simulink model "switchmodel"  (R2019a)
settings: Solver=FixedStepAuto  StartTime=0.0  StopTime=50  FixedStep=1  RelTol=1e-3
settings Model: Creator=anton  LastModifiedBy=anton

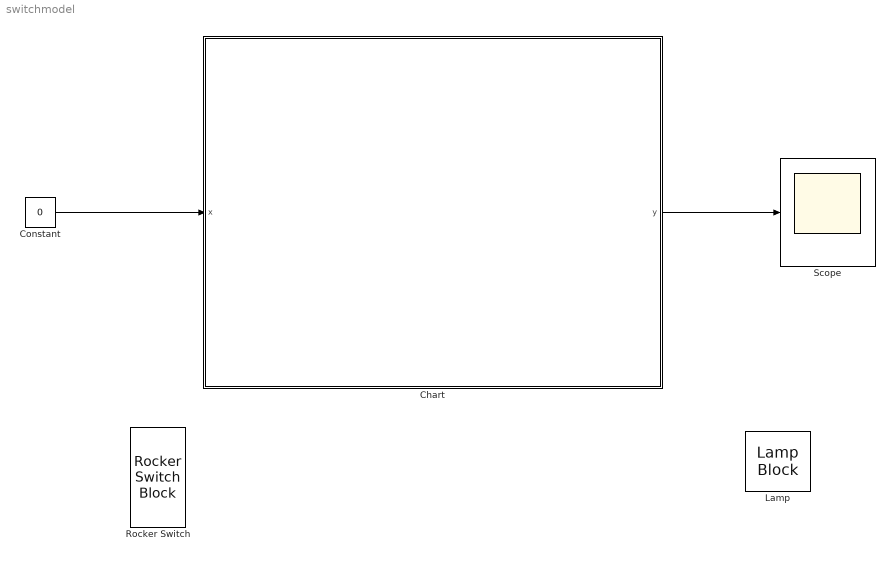
== system switchmodel ==
  Chart : Stateflow chart  BlockKeywords=__PRM__SERIALIZED__DATA__:Stateflow Chart,Stateflow Diagram  TreatAsAtomicUnit=on
  Constant : Constant  Value=0
  Lamp : LampBlock
  Rocker Switch : RockerSwitchBlock
      settings: Values={{'Off', 'On'}, [0 1]}
  Scope : Scope
  wires:
  Constant/1 -> Chart/1(x)
  Chart/1(y) -> Scope/1

== stateflow chart switchmodel/Chart ==
  state RedON
    y=x;
  state RedOFF
    y=1;
  (default) -> RedON
  RedON -> RedOFF : [after(5,sec)]
  RedOFF -> RedON : [after(15,sec)]
  data: x input; y output
